simulink model "CP_SD_SFC_Lin_b_9558292"  (R2018a)
settings: Solver=ode4  StartTime=0.0  StopTime=3  FixedStep=0.001  RelTol=1e-3
values from neighbouring files (symbols this model uses):
  Ab = [0,0,1,0;0,0,0,1;0,-m*g/Mc,0,0;0,-g*(Mc+m)/(l*Mc),0,0]    [CP_DTSFC_Lin_b_MainFile_9558292.m]
  Bb = [0;0;1/Mc;1/(l*Mc)]    [CP_DTSFC_Lin_b_MainFile_9558292.m]
  Cb = eye(4)    [CP_DTSFC_Lin_b_MainFile_9558292.m]
  Db = zeros(4,1)    [CP_DTSFC_Lin_b_MainFile_9558292.m]
  K_b = K_db    [CP_DTSFC_Lin_b_MainFile_9558292.m]
  x10 = 0.2    [CP_DTSFC_Lin_a_MainFile_n9558292.m]    (also in CP_DTSFC_Lin_b_MainFile_9558292.m)
  x20 = deg2rad(20)    [CP_DTSFC_Lin_a_MainFile_n9558292.m]    (also in CP_DTSFC_Lin_b_MainFile_9558292.m)
  x30 = 0    [CP_DTSFC_Lin_a_MainFile_n9558292.m]    (also in CP_DTSFC_Lin_b_MainFile_9558292.m)
  x40 = 0    [CP_DTSFC_Lin_a_MainFile_n9558292.m]    (also in CP_DTSFC_Lin_b_MainFile_9558292.m)
settings Model: Creator=haidarobeid  LastModifiedBy=haidarobeid

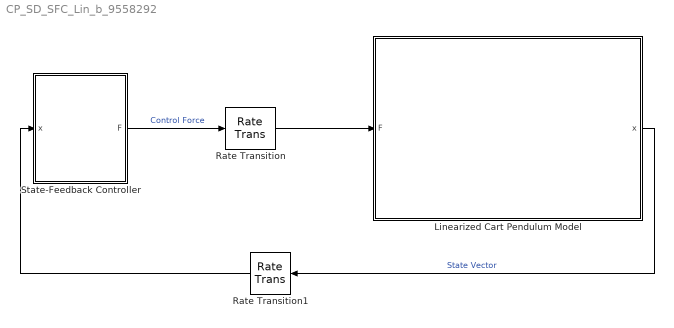
== system CP_SD_SFC_Lin_b_9558292 ==
  Linearized Cart Pendulum Model : Subsystem
  Rate Transition : RateTransition  InitialCondition=-K_b*[x10;x20;x30;x40]
  Rate Transition1 : RateTransition  InitialCondition=[x10;x20;x30;x40]  OutPortSampleTime=T_s
  State-Feedback Controller : Subsystem
  wires:
  State-Feedback Controller/1(F) -> Rate Transition/1  "Control Force"
  Linearized Cart Pendulum Model/1(x) -> Rate Transition1/1  "State Vector"
  Rate Transition/1 -> Linearized Cart Pendulum Model/1(F)
  Rate Transition1/1 -> State-Feedback Controller/1(x)

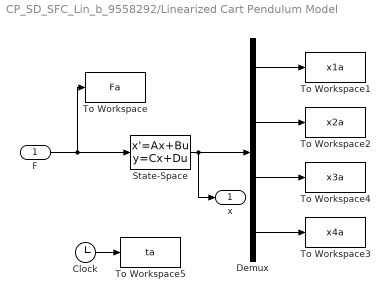
== system CP_SD_SFC_Lin_b_9558292/Linearized Cart Pendulum Model ==
  F : Inport
  Clock : Clock
  Demux : Demux
  State-Space : StateSpace  A=Ab  B=Bb  C=Cb  D=Db  InitialCondition=[x10;x20;x30;x40]
  To Workspace : ToWorkspace  VariableName=Fa  SampleTime=-1
  To Workspace1 : ToWorkspace  VariableName=x1a  SampleTime=-1
  To Workspace2 : ToWorkspace  VariableName=x2a  SampleTime=-1
  To Workspace3 : ToWorkspace  VariableName=x4a  SampleTime=-1
  To Workspace4 : ToWorkspace  VariableName=x3a  SampleTime=-1
  To Workspace5 : ToWorkspace  VariableName=ta  SampleTime=-1
  x : Outport
  wires:
  Demux/3 -> To Workspace4/1
  Demux/2 -> To Workspace2/1
  Demux/4 -> To Workspace3/1
  State-Space/1 -> Demux/1, x/1
  F/1 -> To Workspace/1, State-Space/1
  Demux/1 -> To Workspace1/1
  Clock/1 -> To Workspace5/1

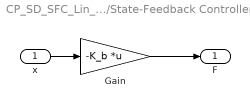
== system CP_SD_SFC_Lin_b_9558292/State-Feedback Controller ==
  x : Inport
  Gain : Gain  Gain=-K_b  Multiplication=Matrix(K*u)
  F : Outport
  wires:
  Gain/1 -> F/1
  x/1 -> Gain/1
